simulink model "helicopter_control"  (R2017a)
settings: Solver=VariableStepAuto  StartTime=0.0  StopTime=100  RelTol=1e-3
settings Model: Creator=mrsmash  LastModifiedBy=mrsmash

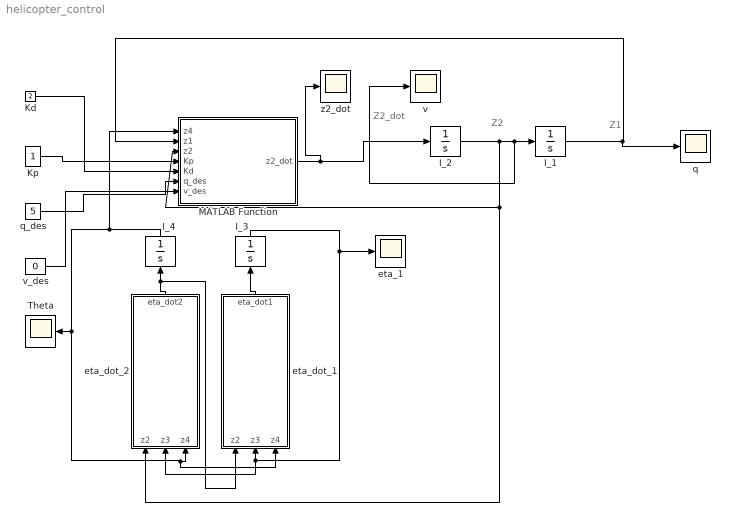
== system helicopter_control ==
  note: Z2_dot
  note: Z1
  note: Z2
  I_1 : Integrator  InitialCondition=5
  I_2 : Integrator
  I_3 : Integrator
  I_4 : Integrator
  Kd : Constant  Value=2
  Kp : Constant
  MATLAB Function : MATLAB Function  TreatAsAtomicUnit=on
  Theta : Scope
  eta_1 : Scope
  eta_dot_1 : MATLAB Function  TreatAsAtomicUnit=on
  eta_dot_2 : MATLAB Function  TreatAsAtomicUnit=on
  q : Scope
  q_des : Constant  Value=5
  v : Scope
  v_des : Constant  Value=0
  z2_dot : Scope
  wires:
  I_2/1 -> MATLAB Function/3(z2), eta_dot_2/1(z2), v/1, I_1/1
  I_1/1 -> q/1, MATLAB Function/2(z1)
  MATLAB Function/1(z2_dot) -> z2_dot/1, I_2/1
  eta_dot_2/1(eta_dot2) -> eta_dot_1/1(z2), I_4/1
  eta_dot_1/1(eta_dot1) -> I_3/1
  I_4/1 -> MATLAB Function/1(z4), Theta/1, eta_dot_1/3(z4), eta_dot_2/3(z4)
  I_3/1 -> eta_1/1, eta_dot_2/2(z3), eta_dot_1/2(z3)
  Kp/1 -> MATLAB Function/4(Kp)
  Kd/1 -> MATLAB Function/5(Kd)
  q_des/1 -> MATLAB Function/6(q_des)
  v_des/1 -> MATLAB Function/7(v_des)

== matlab function helicopter_control/eta_dot_2 ==
  data: z2 input; eta_dot2 output; z3 input; z4 input
function eta_dot2 = eta_dot_2(z2,z3,z4)
g = 9.81;
L = 10;
M = 10;


eta_dot2 =  (z3-z2*L)*M*cos(z4);
end

== matlab function helicopter_control/eta_dot_1 ==
  data: z2 input; z3 input; z4 input; eta_dot1 output
function eta_dot1 = eta_dot_1(z2,z3, z4)

g = 9.81;
L = 10;
M = 10;


eta_dot1 = tan(z4)*(-g*L+z3-z2*L);

end

== matlab function helicopter_control/MATLAB Function ==
  data: z4 input; z1 input; z2 input; z2_dot output; Kp input; Kd input; q_des input; v_des input
function z2_dot = contoller(z4,z1,z2,Kp,Kd,q_des,v_des)

g = 9.81;
L = 10;
M = 10;

v = Kp*(q_des - z1)+Kd*(v_des-z2);
z2_dot = (-g*L*tan(z4)+v)*M*cos(z4);
end
